simulink model "Basics"  (R2019a)
settings: Solver=ode1  StartTime=0.0  StopTime=2.5  FixedStep=Ts_Power  RelTol=1e-3
PostLoadFcn:
  | %% Init for wind PnO models - global system parameters
  | OVERRIDE_SSN_MEMORY_LIMIT=1;
  | Ts=50e-6;
  | % Ts=50e-10;
  | Ts_Power=Ts;
  | Ts_Control=2*Ts;
  | freq = 50;
  | Fnom=freq;
  | Vac=400e3;
InitFcn:
  | %% Init for wind PnO models - global system parameters
  | OVERRIDE_SSN_MEMORY_LIMIT=1;
  | Ts=50e-6;
  | % Ts=50e-10;
  | Ts_Power=Ts;
  | Ts_Control=2*Ts;
  | freq = 50;
  | Fnom=freq;
  | Vac=225e3;
values from neighbouring files (symbols this model uses):
  ohl_posCap = 11.33e-009/2    (= 5.665e-09)    [variable.m]
  ohl_posInd = 1.05e-3/2    (= 0.000525)    [variable.m]
  ohl_posR = 0.1153/2    (= 0.05765)    [variable.m]
  ohl_zeroCap = 5.01e-009/2    (= 2.505e-09)    [variable.m]
  ohl_zeroInd = 3.32e-3/2    (= 0.00166)    [variable.m]
  ohl_zeroR = 0.4138/2    (= 0.2069)    [variable.m]
  sub_posCap = 0.16e-006    (= 1.6e-07)    [variable.m]
  sub_posInd = 0.001400563    [variable.m]
  sub_posR = 0.036    [variable.m]
  sub_zeroCap = 0.053333e-006    (= 5.3333e-08)    [variable.m]
  sub_zeroInd = 0.00420169    [variable.m]
  sub_zeroR = 0.108    [variable.m]
  transfo_L1 = 0.05999374    [variable.m]
  transfo_L2 = 0.05999374    [variable.m]
  transfo_R1 = 0.000866667    [variable.m]
  transfo_R2 = 0.00086667    [variable.m]
undefined symbols (not defined in the file or in its folder): D1, D11, Delta, den, DiscIntNeverNeededParam, dx, find_system, gcbh, num, out_Buses, out_WindFarms, sps_rtmsupport
libraries: powerlib x173, simulink x80, powerlib_meascontrol x80, elements x52, eeSinusoidalMeasurement x46, simulink_extras x40, spsVIMeasurementModel x36, eePowerMeasurement x15
(part 14 of 22)

== system Basics/SM_WT1/Differential Element 1/Main Protection (Current Differential)/Charging Current Compensation phase A/DAB7 ==
  a : Inport
  AD & Buffer : S-Function  FunctionName=dab2  Parameters=winsize,fs,dx,resdis  SFunctionDeploymentMode=off  EnableBusSupport=off
  Analog Filter : TransferFcn  Numerator=num  Denominator=den
  Gain : Gain  Gain=G  SaturateOnIntegerOverflow=on  OutDataTypeStr=Inherit: Same as input  ParamDataTypeStr=Inherit: Same as input
  Zero-Order Hold : ZeroOrderHold  SampleTime=1/fs
  d : Outport  InitialOutput=[zeros(winsize,1)]  VectorParamsAs1DForOutWhenUnconnected=on
  wires:
  AD & Buffer/1 -> d/1
  a/1 -> Analog Filter/1
  Zero-Order Hold/1 -> AD & Buffer/1
  Gain/1 -> Zero-Order Hold/1
  Analog Filter/1 -> Gain/1

== system Basics/SM_WT1/Differential Element 1/Main Protection (Current Differential)/Charging Current Compensation phase B/DAB5 ==
  a : Inport
  AD & Buffer : S-Function  FunctionName=dab2  Parameters=winsize,fs,dx,resdis  SFunctionDeploymentMode=off  EnableBusSupport=off
  Analog Filter : TransferFcn  Numerator=num  Denominator=den
  Gain : Gain  Gain=G  SaturateOnIntegerOverflow=on  OutDataTypeStr=Inherit: Same as input  ParamDataTypeStr=Inherit: Same as input
  Zero-Order Hold : ZeroOrderHold  SampleTime=1/fs
  d : Outport  InitialOutput=[zeros(winsize,1)]  VectorParamsAs1DForOutWhenUnconnected=on
  wires:
  AD & Buffer/1 -> d/1
  a/1 -> Analog Filter/1
  Zero-Order Hold/1 -> AD & Buffer/1
  Gain/1 -> Zero-Order Hold/1
  Analog Filter/1 -> Gain/1

== system Basics/SM_WT1/Differential Element 1/Main Protection (Current Differential)/Charging Current Compensation phase B/DAB6 ==
  a : Inport
  AD & Buffer : S-Function  FunctionName=dab2  Parameters=winsize,fs,dx,resdis  SFunctionDeploymentMode=off  EnableBusSupport=off
  Analog Filter : TransferFcn  Numerator=num  Denominator=den
  Gain : Gain  Gain=G  SaturateOnIntegerOverflow=on  OutDataTypeStr=Inherit: Same as input  ParamDataTypeStr=Inherit: Same as input
  Zero-Order Hold : ZeroOrderHold  SampleTime=1/fs
  d : Outport  InitialOutput=[zeros(winsize,1)]  VectorParamsAs1DForOutWhenUnconnected=on
  wires:
  Analog Filter/1 -> Gain/1
  Gain/1 -> Zero-Order Hold/1
  Zero-Order Hold/1 -> AD & Buffer/1
  a/1 -> Analog Filter/1
  AD & Buffer/1 -> d/1

== system Basics/SM_WT1/Differential Element 1/Main Protection (Current Differential)/Charging Current Compensation phase B/DAB7 ==
  a : Inport
  AD & Buffer : S-Function  FunctionName=dab2  Parameters=winsize,fs,dx,resdis  SFunctionDeploymentMode=off  EnableBusSupport=off
  Analog Filter : TransferFcn  Numerator=num  Denominator=den
  Gain : Gain  Gain=G  SaturateOnIntegerOverflow=on  OutDataTypeStr=Inherit: Same as input  ParamDataTypeStr=Inherit: Same as input
  Zero-Order Hold : ZeroOrderHold  SampleTime=1/fs
  d : Outport  InitialOutput=[zeros(winsize,1)]  VectorParamsAs1DForOutWhenUnconnected=on
  wires:
  AD & Buffer/1 -> d/1
  a/1 -> Analog Filter/1
  Zero-Order Hold/1 -> AD & Buffer/1
  Gain/1 -> Zero-Order Hold/1
  Analog Filter/1 -> Gain/1

== system Basics/SM_WT1/Differential Element 1/Main Protection (Current Differential)/Charging Current Compensation phase C/DAB5 ==
  a : Inport
  AD & Buffer : S-Function  FunctionName=dab2  Parameters=winsize,fs,dx,resdis  SFunctionDeploymentMode=off  EnableBusSupport=off
  Analog Filter : TransferFcn  Numerator=num  Denominator=den
  Gain : Gain  Gain=G  SaturateOnIntegerOverflow=on  OutDataTypeStr=Inherit: Same as input  ParamDataTypeStr=Inherit: Same as input
  Zero-Order Hold : ZeroOrderHold  SampleTime=1/fs
  d : Outport  InitialOutput=[zeros(winsize,1)]  VectorParamsAs1DForOutWhenUnconnected=on
  wires:
  AD & Buffer/1 -> d/1
  a/1 -> Analog Filter/1
  Zero-Order Hold/1 -> AD & Buffer/1
  Gain/1 -> Zero-Order Hold/1
  Analog Filter/1 -> Gain/1

== system Basics/SM_WT1/Differential Element 1/Main Protection (Current Differential)/Charging Current Compensation phase C/DAB6 ==
  a : Inport
  AD & Buffer : S-Function  FunctionName=dab2  Parameters=winsize,fs,dx,resdis  SFunctionDeploymentMode=off  EnableBusSupport=off
  Analog Filter : TransferFcn  Numerator=num  Denominator=den
  Gain : Gain  Gain=G  SaturateOnIntegerOverflow=on  OutDataTypeStr=Inherit: Same as input  ParamDataTypeStr=Inherit: Same as input
  Zero-Order Hold : ZeroOrderHold  SampleTime=1/fs
  d : Outport  InitialOutput=[zeros(winsize,1)]  VectorParamsAs1DForOutWhenUnconnected=on
  wires:
  Analog Filter/1 -> Gain/1
  Gain/1 -> Zero-Order Hold/1
  Zero-Order Hold/1 -> AD & Buffer/1
  a/1 -> Analog Filter/1
  AD & Buffer/1 -> d/1

== system Basics/SM_WT1/Differential Element 1/Main Protection (Current Differential)/Charging Current Compensation phase C/DAB7 ==
  a : Inport
  AD & Buffer : S-Function  FunctionName=dab2  Parameters=winsize,fs,dx,resdis  SFunctionDeploymentMode=off  EnableBusSupport=off
  Analog Filter : TransferFcn  Numerator=num  Denominator=den
  Gain : Gain  Gain=G  SaturateOnIntegerOverflow=on  OutDataTypeStr=Inherit: Same as input  ParamDataTypeStr=Inherit: Same as input
  Zero-Order Hold : ZeroOrderHold  SampleTime=1/fs
  d : Outport  InitialOutput=[zeros(winsize,1)]  VectorParamsAs1DForOutWhenUnconnected=on
  wires:
  AD & Buffer/1 -> d/1
  a/1 -> Analog Filter/1
  Zero-Order Hold/1 -> AD & Buffer/1
  Gain/1 -> Zero-Order Hold/1
  Analog Filter/1 -> Gain/1

== system Basics/SM_WT1/Differential Element 1/Main Protection (Current Differential)/Current Differential Protection for Phase A/Comparision Scheme ==
  I_Slave : Inport
  I_Master : Inport  Port=2
  Abs : Abs  SaturateOnIntegerOverflow=on
  Abs1 : Abs  SaturateOnIntegerOverflow=on
  Bias Characteristic1 : elements/Bias Characteristic  BC=bias  fs=Freq*20
  "Differential Current " : Sum  SaturateOnIntegerOverflow=on  InputSameDT=on  OutDataTypeStr=Inherit: Same as first input
  Restraining Current : Sum  Inputs=+-  SaturateOnIntegerOverflow=on  InputSameDT=on  OutDataTypeStr=Inherit: Same as first input
  Pickup : Outport  VectorParamsAs1DForOutWhenUnconnected=on
  wires:
  "Differential Current "/1 -> Abs/1
  Abs1/1 -> Bias Characteristic1/2
  Bias Characteristic1/1 -> Pickup/1
  Abs/1 -> Bias Characteristic1/1
  I_Master/1 -> Restraining Current/2, "Differential Current "/2
  I_Slave/1 -> Restraining Current/1, "Differential Current "/1
  Restraining Current/1 -> Abs1/1

== system Basics/SM_WT1/Differential Element 1/Main Protection (Current Differential)/Current Differential Protection for Phase A/DAB4 ==
  a : Inport
  AD & Buffer : S-Function  FunctionName=dab2  Parameters=winsize,fs,dx,resdis  SFunctionDeploymentMode=off  EnableBusSupport=off
  Analog Filter : TransferFcn  Numerator=num  Denominator=den
  Gain : Gain  Gain=G  SaturateOnIntegerOverflow=on  OutDataTypeStr=Inherit: Same as input  ParamDataTypeStr=Inherit: Same as input
  Zero-Order Hold : ZeroOrderHold  SampleTime=1/fs
  d : Outport  InitialOutput=[zeros(winsize,1)]  VectorParamsAs1DForOutWhenUnconnected=on
  wires:
  AD & Buffer/1 -> d/1
  a/1 -> Analog Filter/1
  Zero-Order Hold/1 -> AD & Buffer/1
  Gain/1 -> Zero-Order Hold/1
  Analog Filter/1 -> Gain/1

== system Basics/SM_WT1/Differential Element 1/Main Protection (Current Differential)/Current Differential Protection for Phase A/DAB8 ==
  a : Inport
  AD & Buffer : S-Function  FunctionName=dab2  Parameters=winsize,fs,dx,resdis  SFunctionDeploymentMode=off  EnableBusSupport=off
  Analog Filter : TransferFcn  Numerator=num  Denominator=den
  Gain : Gain  Gain=G  SaturateOnIntegerOverflow=on  OutDataTypeStr=Inherit: Same as input  ParamDataTypeStr=Inherit: Same as input
  Zero-Order Hold : ZeroOrderHold  SampleTime=1/fs
  d : Outport  InitialOutput=[zeros(winsize,1)]  VectorParamsAs1DForOutWhenUnconnected=on
  wires:
  Analog Filter/1 -> Gain/1
  Gain/1 -> Zero-Order Hold/1
  Zero-Order Hold/1 -> AD & Buffer/1
  a/1 -> Analog Filter/1
  AD & Buffer/1 -> d/1

== system Basics/SM_WT1/Differential Element 1/Main Protection (Current Differential)/Current Differential Protection for Phase B/Comparision Scheme ==
  I_Slave : Inport
  I_Master : Inport  Port=2
  Abs : Abs  SaturateOnIntegerOverflow=on
  Abs1 : Abs  SaturateOnIntegerOverflow=on
  Bias Characteristic1 : elements/Bias Characteristic  BC=bias  fs=Freq*20
  "Differential Current " : Sum  SaturateOnIntegerOverflow=on  InputSameDT=on  OutDataTypeStr=Inherit: Same as first input
  Restraining Current : Sum  Inputs=+-  SaturateOnIntegerOverflow=on  InputSameDT=on  OutDataTypeStr=Inherit: Same as first input
  Pickup : Outport  VectorParamsAs1DForOutWhenUnconnected=on
  wires:
  Restraining Current/1 -> Abs1/1
  I_Slave/1 -> "Differential Current "/1, Restraining Current/1
  I_Master/1 -> "Differential Current "/2, Restraining Current/2
  Abs/1 -> Bias Characteristic1/1
  Bias Characteristic1/1 -> Pickup/1
  Abs1/1 -> Bias Characteristic1/2
  "Differential Current "/1 -> Abs/1

== system Basics/SM_WT1/Differential Element 1/Main Protection (Current Differential)/Current Differential Protection for Phase B/DAB4 ==
  a : Inport
  AD & Buffer : S-Function  FunctionName=dab2  Parameters=winsize,fs,dx,resdis  SFunctionDeploymentMode=off  EnableBusSupport=off
  Analog Filter : TransferFcn  Numerator=num  Denominator=den
  Gain : Gain  Gain=G  SaturateOnIntegerOverflow=on  OutDataTypeStr=Inherit: Same as input  ParamDataTypeStr=Inherit: Same as input
  Zero-Order Hold : ZeroOrderHold  SampleTime=1/fs
  d : Outport  InitialOutput=[zeros(winsize,1)]  VectorParamsAs1DForOutWhenUnconnected=on
  wires:
  Analog Filter/1 -> Gain/1
  Gain/1 -> Zero-Order Hold/1
  Zero-Order Hold/1 -> AD & Buffer/1
  a/1 -> Analog Filter/1
  AD & Buffer/1 -> d/1

== system Basics/SM_WT1/Differential Element 1/Main Protection (Current Differential)/Current Differential Protection for Phase B/DAB8 ==
  a : Inport
  AD & Buffer : S-Function  FunctionName=dab2  Parameters=winsize,fs,dx,resdis  SFunctionDeploymentMode=off  EnableBusSupport=off
  Analog Filter : TransferFcn  Numerator=num  Denominator=den
  Gain : Gain  Gain=G  SaturateOnIntegerOverflow=on  OutDataTypeStr=Inherit: Same as input  ParamDataTypeStr=Inherit: Same as input
  Zero-Order Hold : ZeroOrderHold  SampleTime=1/fs
  d : Outport  InitialOutput=[zeros(winsize,1)]  VectorParamsAs1DForOutWhenUnconnected=on
  wires:
  AD & Buffer/1 -> d/1
  a/1 -> Analog Filter/1
  Zero-Order Hold/1 -> AD & Buffer/1
  Gain/1 -> Zero-Order Hold/1
  Analog Filter/1 -> Gain/1

== system Basics/SM_WT1/Differential Element 1/Main Protection (Current Differential)/Current Differential Protection for Phase C/Comparision Scheme ==
  I_Slave : Inport
  I_Master : Inport  Port=2
  Abs : Abs  SaturateOnIntegerOverflow=on
  Abs1 : Abs  SaturateOnIntegerOverflow=on
  Bias Characteristic1 : elements/Bias Characteristic  BC=bias  fs=Freq*20
  "Differential Current " : Sum  SaturateOnIntegerOverflow=on  InputSameDT=on  OutDataTypeStr=Inherit: Same as first input
  Restraining Current : Sum  Inputs=+-  SaturateOnIntegerOverflow=on  InputSameDT=on  OutDataTypeStr=Inherit: Same as first input
  Pickup : Outport  VectorParamsAs1DForOutWhenUnconnected=on
  wires:
  "Differential Current "/1 -> Abs/1
  Abs1/1 -> Bias Characteristic1/2
  Bias Characteristic1/1 -> Pickup/1
  Abs/1 -> Bias Characteristic1/1
  I_Master/1 -> Restraining Current/2, "Differential Current "/2
  I_Slave/1 -> Restraining Current/1, "Differential Current "/1
  Restraining Current/1 -> Abs1/1

== system Basics/SM_WT1/Differential Element 1/Main Protection (Current Differential)/Current Differential Protection for Phase C/DAB4 ==
  a : Inport
  AD & Buffer : S-Function  FunctionName=dab2  Parameters=winsize,fs,dx,resdis  SFunctionDeploymentMode=off  EnableBusSupport=off
  Analog Filter : TransferFcn  Numerator=num  Denominator=den
  Gain : Gain  Gain=G  SaturateOnIntegerOverflow=on  OutDataTypeStr=Inherit: Same as input  ParamDataTypeStr=Inherit: Same as input
  Zero-Order Hold : ZeroOrderHold  SampleTime=1/fs
  d : Outport  InitialOutput=[zeros(winsize,1)]  VectorParamsAs1DForOutWhenUnconnected=on
  wires:
  AD & Buffer/1 -> d/1
  a/1 -> Analog Filter/1
  Zero-Order Hold/1 -> AD & Buffer/1
  Gain/1 -> Zero-Order Hold/1
  Analog Filter/1 -> Gain/1

== system Basics/SM_WT1/Differential Element 1/Main Protection (Current Differential)/Current Differential Protection for Phase C/DAB8 ==
  a : Inport
  AD & Buffer : S-Function  FunctionName=dab2  Parameters=winsize,fs,dx,resdis  SFunctionDeploymentMode=off  EnableBusSupport=off
  Analog Filter : TransferFcn  Numerator=num  Denominator=den
  Gain : Gain  Gain=G  SaturateOnIntegerOverflow=on  OutDataTypeStr=Inherit: Same as input  ParamDataTypeStr=Inherit: Same as input
  Zero-Order Hold : ZeroOrderHold  SampleTime=1/fs
  d : Outport  InitialOutput=[zeros(winsize,1)]  VectorParamsAs1DForOutWhenUnconnected=on
  wires:
  Analog Filter/1 -> Gain/1
  Gain/1 -> Zero-Order Hold/1
  Zero-Order Hold/1 -> AD & Buffer/1
  a/1 -> Analog Filter/1
  AD & Buffer/1 -> d/1

== system Basics/SM_WT1/Differential Element 2/Main Protection (Current Differential)/Charging Current Compensation phase A/DAB5 ==
  a : Inport
  AD & Buffer : S-Function  FunctionName=dab2  Parameters=winsize,fs,dx,resdis  SFunctionDeploymentMode=off  EnableBusSupport=off
  Analog Filter : TransferFcn  Numerator=num  Denominator=den
  Gain : Gain  Gain=G  SaturateOnIntegerOverflow=on  OutDataTypeStr=Inherit: Same as input  ParamDataTypeStr=Inherit: Same as input
  Zero-Order Hold : ZeroOrderHold  SampleTime=1/fs
  d : Outport  InitialOutput=[zeros(winsize,1)]  VectorParamsAs1DForOutWhenUnconnected=on
  wires:
  AD & Buffer/1 -> d/1
  a/1 -> Analog Filter/1
  Zero-Order Hold/1 -> AD & Buffer/1
  Gain/1 -> Zero-Order Hold/1
  Analog Filter/1 -> Gain/1

== system Basics/SM_WT1/Differential Element 2/Main Protection (Current Differential)/Charging Current Compensation phase A/DAB6 ==
  a : Inport
  AD & Buffer : S-Function  FunctionName=dab2  Parameters=winsize,fs,dx,resdis  SFunctionDeploymentMode=off  EnableBusSupport=off
  Analog Filter : TransferFcn  Numerator=num  Denominator=den
  Gain : Gain  Gain=G  SaturateOnIntegerOverflow=on  OutDataTypeStr=Inherit: Same as input  ParamDataTypeStr=Inherit: Same as input
  Zero-Order Hold : ZeroOrderHold  SampleTime=1/fs
  d : Outport  InitialOutput=[zeros(winsize,1)]  VectorParamsAs1DForOutWhenUnconnected=on
  wires:
  Analog Filter/1 -> Gain/1
  Gain/1 -> Zero-Order Hold/1
  Zero-Order Hold/1 -> AD & Buffer/1
  a/1 -> Analog Filter/1
  AD & Buffer/1 -> d/1

== system Basics/SM_WT1/Differential Element 2/Main Protection (Current Differential)/Charging Current Compensation phase A/DAB7 ==
  a : Inport
  AD & Buffer : S-Function  FunctionName=dab2  Parameters=winsize,fs,dx,resdis  SFunctionDeploymentMode=off  EnableBusSupport=off
  Analog Filter : TransferFcn  Numerator=num  Denominator=den
  Gain : Gain  Gain=G  SaturateOnIntegerOverflow=on  OutDataTypeStr=Inherit: Same as input  ParamDataTypeStr=Inherit: Same as input
  Zero-Order Hold : ZeroOrderHold  SampleTime=1/fs
  d : Outport  InitialOutput=[zeros(winsize,1)]  VectorParamsAs1DForOutWhenUnconnected=on
  wires:
  AD & Buffer/1 -> d/1
  a/1 -> Analog Filter/1
  Zero-Order Hold/1 -> AD & Buffer/1
  Gain/1 -> Zero-Order Hold/1
  Analog Filter/1 -> Gain/1

== system Basics/SM_WT1/Differential Element 2/Main Protection (Current Differential)/Charging Current Compensation phase B/DAB5 ==
  a : Inport
  AD & Buffer : S-Function  FunctionName=dab2  Parameters=winsize,fs,dx,resdis  SFunctionDeploymentMode=off  EnableBusSupport=off
  Analog Filter : TransferFcn  Numerator=num  Denominator=den
  Gain : Gain  Gain=G  SaturateOnIntegerOverflow=on  OutDataTypeStr=Inherit: Same as input  ParamDataTypeStr=Inherit: Same as input
  Zero-Order Hold : ZeroOrderHold  SampleTime=1/fs
  d : Outport  InitialOutput=[zeros(winsize,1)]  VectorParamsAs1DForOutWhenUnconnected=on
  wires:
  AD & Buffer/1 -> d/1
  a/1 -> Analog Filter/1
  Zero-Order Hold/1 -> AD & Buffer/1
  Gain/1 -> Zero-Order Hold/1
  Analog Filter/1 -> Gain/1

== system Basics/SM_WT1/Differential Element 2/Main Protection (Current Differential)/Charging Current Compensation phase B/DAB6 ==
  a : Inport
  AD & Buffer : S-Function  FunctionName=dab2  Parameters=winsize,fs,dx,resdis  SFunctionDeploymentMode=off  EnableBusSupport=off
  Analog Filter : TransferFcn  Numerator=num  Denominator=den
  Gain : Gain  Gain=G  SaturateOnIntegerOverflow=on  OutDataTypeStr=Inherit: Same as input  ParamDataTypeStr=Inherit: Same as input
  Zero-Order Hold : ZeroOrderHold  SampleTime=1/fs
  d : Outport  InitialOutput=[zeros(winsize,1)]  VectorParamsAs1DForOutWhenUnconnected=on
  wires:
  Analog Filter/1 -> Gain/1
  Gain/1 -> Zero-Order Hold/1
  Zero-Order Hold/1 -> AD & Buffer/1
  a/1 -> Analog Filter/1
  AD & Buffer/1 -> d/1

== system Basics/SM_WT1/Differential Element 2/Main Protection (Current Differential)/Charging Current Compensation phase B/DAB7 ==
  a : Inport
  AD & Buffer : S-Function  FunctionName=dab2  Parameters=winsize,fs,dx,resdis  SFunctionDeploymentMode=off  EnableBusSupport=off
  Analog Filter : TransferFcn  Numerator=num  Denominator=den
  Gain : Gain  Gain=G  SaturateOnIntegerOverflow=on  OutDataTypeStr=Inherit: Same as input  ParamDataTypeStr=Inherit: Same as input
  Zero-Order Hold : ZeroOrderHold  SampleTime=1/fs
  d : Outport  InitialOutput=[zeros(winsize,1)]  VectorParamsAs1DForOutWhenUnconnected=on
  wires:
  AD & Buffer/1 -> d/1
  a/1 -> Analog Filter/1
  Zero-Order Hold/1 -> AD & Buffer/1
  Gain/1 -> Zero-Order Hold/1
  Analog Filter/1 -> Gain/1

== system Basics/SM_WT1/Differential Element 2/Main Protection (Current Differential)/Charging Current Compensation phase C/DAB5 ==
  a : Inport
  AD & Buffer : S-Function  FunctionName=dab2  Parameters=winsize,fs,dx,resdis  SFunctionDeploymentMode=off  EnableBusSupport=off
  Analog Filter : TransferFcn  Numerator=num  Denominator=den
  Gain : Gain  Gain=G  SaturateOnIntegerOverflow=on  OutDataTypeStr=Inherit: Same as input  ParamDataTypeStr=Inherit: Same as input
  Zero-Order Hold : ZeroOrderHold  SampleTime=1/fs
  d : Outport  InitialOutput=[zeros(winsize,1)]  VectorParamsAs1DForOutWhenUnconnected=on
  wires:
  AD & Buffer/1 -> d/1
  a/1 -> Analog Filter/1
  Zero-Order Hold/1 -> AD & Buffer/1
  Gain/1 -> Zero-Order Hold/1
  Analog Filter/1 -> Gain/1

== system Basics/SM_WT1/Differential Element 2/Main Protection (Current Differential)/Charging Current Compensation phase C/DAB6 ==
  a : Inport
  AD & Buffer : S-Function  FunctionName=dab2  Parameters=winsize,fs,dx,resdis  SFunctionDeploymentMode=off  EnableBusSupport=off
  Analog Filter : TransferFcn  Numerator=num  Denominator=den
  Gain : Gain  Gain=G  SaturateOnIntegerOverflow=on  OutDataTypeStr=Inherit: Same as input  ParamDataTypeStr=Inherit: Same as input
  Zero-Order Hold : ZeroOrderHold  SampleTime=1/fs
  d : Outport  InitialOutput=[zeros(winsize,1)]  VectorParamsAs1DForOutWhenUnconnected=on
  wires:
  Analog Filter/1 -> Gain/1
  Gain/1 -> Zero-Order Hold/1
  Zero-Order Hold/1 -> AD & Buffer/1
  a/1 -> Analog Filter/1
  AD & Buffer/1 -> d/1

== system Basics/SM_WT1/Differential Element 2/Main Protection (Current Differential)/Charging Current Compensation phase C/DAB7 ==
  a : Inport
  AD & Buffer : S-Function  FunctionName=dab2  Parameters=winsize,fs,dx,resdis  SFunctionDeploymentMode=off  EnableBusSupport=off
  Analog Filter : TransferFcn  Numerator=num  Denominator=den
  Gain : Gain  Gain=G  SaturateOnIntegerOverflow=on  OutDataTypeStr=Inherit: Same as input  ParamDataTypeStr=Inherit: Same as input
  Zero-Order Hold : ZeroOrderHold  SampleTime=1/fs
  d : Outport  InitialOutput=[zeros(winsize,1)]  VectorParamsAs1DForOutWhenUnconnected=on
  wires:
  AD & Buffer/1 -> d/1
  a/1 -> Analog Filter/1
  Zero-Order Hold/1 -> AD & Buffer/1
  Gain/1 -> Zero-Order Hold/1
  Analog Filter/1 -> Gain/1

== system Basics/SM_WT1/Differential Element 2/Main Protection (Current Differential)/Current Differential Protection for Phase A/Comparision Scheme ==
  I_Slave : Inport
  I_Master : Inport  Port=2
  Abs : Abs  SaturateOnIntegerOverflow=on
  Abs1 : Abs  SaturateOnIntegerOverflow=on
  Bias Characteristic1 : elements/Bias Characteristic  BC=bias  fs=Freq*20
  "Differential Current " : Sum  SaturateOnIntegerOverflow=on  InputSameDT=on  OutDataTypeStr=Inherit: Same as first input
  Restraining Current : Sum  Inputs=+-  SaturateOnIntegerOverflow=on  InputSameDT=on  OutDataTypeStr=Inherit: Same as first input
  Pickup : Outport  VectorParamsAs1DForOutWhenUnconnected=on
  wires:
  "Differential Current "/1 -> Abs/1
  Abs1/1 -> Bias Characteristic1/2
  Bias Characteristic1/1 -> Pickup/1
  Abs/1 -> Bias Characteristic1/1
  I_Master/1 -> Restraining Current/2, "Differential Current "/2
  I_Slave/1 -> Restraining Current/1, "Differential Current "/1
  Restraining Current/1 -> Abs1/1

== system Basics/SM_WT1/Differential Element 2/Main Protection (Current Differential)/Current Differential Protection for Phase A/DAB4 ==
  a : Inport
  AD & Buffer : S-Function  FunctionName=dab2  Parameters=winsize,fs,dx,resdis  SFunctionDeploymentMode=off  EnableBusSupport=off
  Analog Filter : TransferFcn  Numerator=num  Denominator=den
  Gain : Gain  Gain=G  SaturateOnIntegerOverflow=on  OutDataTypeStr=Inherit: Same as input  ParamDataTypeStr=Inherit: Same as input
  Zero-Order Hold : ZeroOrderHold  SampleTime=1/fs
  d : Outport  InitialOutput=[zeros(winsize,1)]  VectorParamsAs1DForOutWhenUnconnected=on
  wires:
  AD & Buffer/1 -> d/1
  a/1 -> Analog Filter/1
  Zero-Order Hold/1 -> AD & Buffer/1
  Gain/1 -> Zero-Order Hold/1
  Analog Filter/1 -> Gain/1

== system Basics/SM_WT1/Differential Element 2/Main Protection (Current Differential)/Current Differential Protection for Phase A/DAB8 ==
  a : Inport
  AD & Buffer : S-Function  FunctionName=dab2  Parameters=winsize,fs,dx,resdis  SFunctionDeploymentMode=off  EnableBusSupport=off
  Analog Filter : TransferFcn  Numerator=num  Denominator=den
  Gain : Gain  Gain=G  SaturateOnIntegerOverflow=on  OutDataTypeStr=Inherit: Same as input  ParamDataTypeStr=Inherit: Same as input
  Zero-Order Hold : ZeroOrderHold  SampleTime=1/fs
  d : Outport  InitialOutput=[zeros(winsize,1)]  VectorParamsAs1DForOutWhenUnconnected=on
  wires:
  Analog Filter/1 -> Gain/1
  Gain/1 -> Zero-Order Hold/1
  Zero-Order Hold/1 -> AD & Buffer/1
  a/1 -> Analog Filter/1
  AD & Buffer/1 -> d/1

== system Basics/SM_WT1/Differential Element 2/Main Protection (Current Differential)/Current Differential Protection for Phase B/Comparision Scheme ==
  I_Slave : Inport
  I_Master : Inport  Port=2
  Abs : Abs  SaturateOnIntegerOverflow=on
  Abs1 : Abs  SaturateOnIntegerOverflow=on
  Bias Characteristic1 : elements/Bias Characteristic  BC=bias  fs=Freq*20
  "Differential Current " : Sum  SaturateOnIntegerOverflow=on  InputSameDT=on  OutDataTypeStr=Inherit: Same as first input
  Restraining Current : Sum  Inputs=+-  SaturateOnIntegerOverflow=on  InputSameDT=on  OutDataTypeStr=Inherit: Same as first input
  Pickup : Outport  VectorParamsAs1DForOutWhenUnconnected=on
  wires:
  Restraining Current/1 -> Abs1/1
  I_Slave/1 -> "Differential Current "/1, Restraining Current/1
  I_Master/1 -> "Differential Current "/2, Restraining Current/2
  Abs/1 -> Bias Characteristic1/1
  Bias Characteristic1/1 -> Pickup/1
  Abs1/1 -> Bias Characteristic1/2
  "Differential Current "/1 -> Abs/1

== system Basics/SM_WT1/Differential Element 2/Main Protection (Current Differential)/Current Differential Protection for Phase B/DAB4 ==
  a : Inport
  AD & Buffer : S-Function  FunctionName=dab2  Parameters=winsize,fs,dx,resdis  SFunctionDeploymentMode=off  EnableBusSupport=off
  Analog Filter : TransferFcn  Numerator=num  Denominator=den
  Gain : Gain  Gain=G  SaturateOnIntegerOverflow=on  OutDataTypeStr=Inherit: Same as input  ParamDataTypeStr=Inherit: Same as input
  Zero-Order Hold : ZeroOrderHold  SampleTime=1/fs
  d : Outport  InitialOutput=[zeros(winsize,1)]  VectorParamsAs1DForOutWhenUnconnected=on
  wires:
  Analog Filter/1 -> Gain/1
  Gain/1 -> Zero-Order Hold/1
  Zero-Order Hold/1 -> AD & Buffer/1
  a/1 -> Analog Filter/1
  AD & Buffer/1 -> d/1

== system Basics/SM_WT1/Differential Element 2/Main Protection (Current Differential)/Current Differential Protection for Phase B/DAB8 ==
  a : Inport
  AD & Buffer : S-Function  FunctionName=dab2  Parameters=winsize,fs,dx,resdis  SFunctionDeploymentMode=off  EnableBusSupport=off
  Analog Filter : TransferFcn  Numerator=num  Denominator=den
  Gain : Gain  Gain=G  SaturateOnIntegerOverflow=on  OutDataTypeStr=Inherit: Same as input  ParamDataTypeStr=Inherit: Same as input
  Zero-Order Hold : ZeroOrderHold  SampleTime=1/fs
  d : Outport  InitialOutput=[zeros(winsize,1)]  VectorParamsAs1DForOutWhenUnconnected=on
  wires:
  AD & Buffer/1 -> d/1
  a/1 -> Analog Filter/1
  Zero-Order Hold/1 -> AD & Buffer/1
  Gain/1 -> Zero-Order Hold/1
  Analog Filter/1 -> Gain/1

== system Basics/SM_WT1/Differential Element 2/Main Protection (Current Differential)/Current Differential Protection for Phase C/Comparision Scheme ==
  I_Slave : Inport
  I_Master : Inport  Port=2
  Abs : Abs  SaturateOnIntegerOverflow=on
  Abs1 : Abs  SaturateOnIntegerOverflow=on
  Bias Characteristic1 : elements/Bias Characteristic  BC=bias  fs=Freq*20
  "Differential Current " : Sum  SaturateOnIntegerOverflow=on  InputSameDT=on  OutDataTypeStr=Inherit: Same as first input
  Restraining Current : Sum  Inputs=+-  SaturateOnIntegerOverflow=on  InputSameDT=on  OutDataTypeStr=Inherit: Same as first input
  Pickup : Outport  VectorParamsAs1DForOutWhenUnconnected=on
  wires:
  "Differential Current "/1 -> Abs/1
  Abs1/1 -> Bias Characteristic1/2
  Bias Characteristic1/1 -> Pickup/1
  Abs/1 -> Bias Characteristic1/1
  I_Master/1 -> Restraining Current/2, "Differential Current "/2
  I_Slave/1 -> Restraining Current/1, "Differential Current "/1
  Restraining Current/1 -> Abs1/1

== system Basics/SM_WT1/Differential Element 2/Main Protection (Current Differential)/Current Differential Protection for Phase C/DAB4 ==
  a : Inport
  AD & Buffer : S-Function  FunctionName=dab2  Parameters=winsize,fs,dx,resdis  SFunctionDeploymentMode=off  EnableBusSupport=off
  Analog Filter : TransferFcn  Numerator=num  Denominator=den
  Gain : Gain  Gain=G  SaturateOnIntegerOverflow=on  OutDataTypeStr=Inherit: Same as input  ParamDataTypeStr=Inherit: Same as input
  Zero-Order Hold : ZeroOrderHold  SampleTime=1/fs
  d : Outport  InitialOutput=[zeros(winsize,1)]  VectorParamsAs1DForOutWhenUnconnected=on
  wires:
  AD & Buffer/1 -> d/1
  a/1 -> Analog Filter/1
  Zero-Order Hold/1 -> AD & Buffer/1
  Gain/1 -> Zero-Order Hold/1
  Analog Filter/1 -> Gain/1

== system Basics/SM_WT1/Differential Element 2/Main Protection (Current Differential)/Current Differential Protection for Phase C/DAB8 ==
  a : Inport
  AD & Buffer : S-Function  FunctionName=dab2  Parameters=winsize,fs,dx,resdis  SFunctionDeploymentMode=off  EnableBusSupport=off
  Analog Filter : TransferFcn  Numerator=num  Denominator=den
  Gain : Gain  Gain=G  SaturateOnIntegerOverflow=on  OutDataTypeStr=Inherit: Same as input  ParamDataTypeStr=Inherit: Same as input
  Zero-Order Hold : ZeroOrderHold  SampleTime=1/fs
  d : Outport  InitialOutput=[zeros(winsize,1)]  VectorParamsAs1DForOutWhenUnconnected=on
  wires:
  Analog Filter/1 -> Gain/1
  Gain/1 -> Zero-Order Hold/1
  Zero-Order Hold/1 -> AD & Buffer/1
  a/1 -> Analog Filter/1
  AD & Buffer/1 -> d/1

== system Basics/SM_WT1/Impedance Element 1/Impedance Relay Scheme/Analog filtering, signal conditioning/CURRENTS ==
  Iabc : Inport
  Add : Sum  Inputs=+++
  Complex{,1..3} (4 alike) : MagnitudeAngleToComplex
  Constant : Constant  Value=pi/180
  Constant1 : Constant  Value=k0m1
  Constant2 : Constant  Value=k0a1
  DAB - current A : Subsystem  AncestorBlock=elements/DAB  mask(Data Adquisition Board){filter=off, approx=Butterworth, order=2, numerator=[], denominator=[], freq=fCut, resdis=off, vertres=16, xmax=CurrentRange, winsize=WindowSize, G=1.0, fs=fSampling}
      mask prompts: filter "Disable Analog Filter"; approx "Filter approximation"; numerator "Free expression filter: numerator(descending order of s)"; denominator "Free expression filter: denominator:"; freq "Cut-off frequency"; resdis "Disable Vertical Resolution"; vertres "Vertical Resolution: No. of bits"; xmax "Vertical Resolution: signal range"; winsize "Window size"; G "Gain"; fs "Sampling frequency"
      mask help: Performs analog filtering, signal conditioning and sampling. A single signal is the input, a buffer with the signal samples is the output. The options include analog filter enable/disable switch, type, order and cut-off frequency of the analog filter, conditioning gain, sampling frequency, number of bits, the length of the buffer.
      mask init:
      | dab1
      mask Help: web(['file:///' which('dabdoc2.html')]);
      mask TypeOptions approx: Bessel | Tschebyscheff | Butterworth | free expression
      mask TypeOptions order: 2 | 3 | 4
      mask TypeOptions vertres: 8 | 12 | 16
      mask Display: disp('DAB')
  DAB - current B : Subsystem  AncestorBlock=elements/DAB  mask(Data Adquisition Board){filter=off, approx=Butterworth, order=2, numerator=[], denominator=[], freq=fCut, resdis=off, vertres=16, xmax=CurrentRange, winsize=WindowSize, G=1.0, fs=fSampling}
      mask prompts: filter "Disable Analog Filter"; approx "Filter approximation"; numerator "Free expression filter: numerator(descending order of s)"; denominator "Free expression filter: denominator:"; freq "Cut-off frequency"; resdis "Disable Vertical Resolution"; vertres "Vertical Resolution: No. of bits"; xmax "Vertical Resolution: signal range"; winsize "Window size"; G "Gain"; fs "Sampling frequency"
      mask help: Performs analog filtering, signal conditioning and sampling. A single signal is the input, a buffer with the signal samples is the output. The options include analog filter enable/disable switch, type, order and cut-off frequency of the analog filter, conditioning gain, sampling frequency, number of bits, the length of the buffer.
      mask init:
      | dab1
      mask Help: web(['file:///' which('dabdoc2.html')]);
      mask TypeOptions approx: Bessel | Tschebyscheff | Butterworth | free expression
      mask TypeOptions order: 2 | 3 | 4
      mask TypeOptions vertres: 8 | 12 | 16
      mask Display: disp('DAB')
  DAB - current C : Subsystem  AncestorBlock=elements/DAB  mask(Data Adquisition Board){filter=off, approx=Butterworth, order=2, numerator=[], denominator=[], freq=fCut, resdis=off, vertres=16, xmax=CurrentRange, winsize=WindowSize, G=1.0, fs=fSampling}
      mask prompts: filter "Disable Analog Filter"; approx "Filter approximation"; numerator "Free expression filter: numerator(descending order of s)"; denominator "Free expression filter: denominator:"; freq "Cut-off frequency"; resdis "Disable Vertical Resolution"; vertres "Vertical Resolution: No. of bits"; xmax "Vertical Resolution: signal range"; winsize "Window size"; G "Gain"; fs "Sampling frequency"
      mask help: Performs analog filtering, signal conditioning and sampling. A single signal is the input, a buffer with the signal samples is the output. The options include analog filter enable/disable switch, type, order and cut-off frequency of the analog filter, conditioning gain, sampling frequency, number of bits, the length of the buffer.
      mask init:
      | dab1
      mask Help: web(['file:///' which('dabdoc2.html')]);
      mask TypeOptions approx: Bessel | Tschebyscheff | Butterworth | free expression
      mask TypeOptions order: 2 | 3 | 4
      mask TypeOptions vertres: 8 | 12 | 16
      mask Display: disp('DAB')
  Demux : Demux  Outputs=3
  Phasor IA : Subsystem  AncestorBlock=powerlib_extras/Measurements/Fourier  DialogController=POWERSYS.PowerSysDialog  mask(Fourier analyser){f1=Freq, n=1}
      mask prompts: f1 "Fundamental frequency f1 (Hz):"; n "Harmonic n (0=DC; 1=fundamental; 2=2nd harm;  ...) :"
      mask help: The Fourier block performs a Fourier analysis of the input signal over a running window of one cycle of the fundamental frequency. First and second outputs return respectively the magnitude and phase (degrees) of the harmonic component specified.
      mask init:
      | k=2-(n==0);
      | power_initmask();
      mask Help: web(psbhelp)
  Phasor IB : Subsystem  AncestorBlock=powerlib_extras/Measurements/Fourier  DialogController=POWERSYS.PowerSysDialog  mask(Fourier analyser){f1=Freq, n=1}
      mask prompts: f1 "Fundamental frequency f1 (Hz):"; n "Harmonic n (0=DC; 1=fundamental; 2=2nd harm;  ...) :"
      mask help: The Fourier block performs a Fourier analysis of the input signal over a running window of one cycle of the fundamental frequency. First and second outputs return respectively the magnitude and phase (degrees) of the harmonic component specified.
      mask init:
      | k=2-(n==0);
      | power_initmask();
      mask Help: web(psbhelp)
  Phasor IC : Subsystem  AncestorBlock=powerlib_extras/Measurements/Fourier  DialogController=POWERSYS.PowerSysDialog  mask(Fourier analyser){f1=Freq, n=1}
      mask prompts: f1 "Fundamental frequency f1 (Hz):"; n "Harmonic n (0=DC; 1=fundamental; 2=2nd harm;  ...) :"
      mask help: The Fourier block performs a Fourier analysis of the input signal over a running window of one cycle of the fundamental frequency. First and second outputs return respectively the magnitude and phase (degrees) of the harmonic component specified.
      mask init:
      | k=2-(n==0);
      | power_initmask();
      mask Help: web(psbhelp)
  Product{,1..3,5} (5 alike) : Product  RndMeth=Zero
  IAf : Outport  InitialOutput=0  VectorParamsAs1DForOutWhenUnconnected=on
  IBf : Outport  Port=2  InitialOutput=0  VectorParamsAs1DForOutWhenUnconnected=on
  ICf : Outport  Port=3  InitialOutput=0  VectorParamsAs1DForOutWhenUnconnected=on
  k0I0f : Outport  Port=4  InitialOutput=0  VectorParamsAs1DForOutWhenUnconnected=on
  iaf : Outport  Port=5  InitialOutput=0  VectorParamsAs1DForOutWhenUnconnected=on
  ibf : Outport  Port=6  InitialOutput=0  VectorParamsAs1DForOutWhenUnconnected=on
  icf : Outport  Port=7  InitialOutput=0  VectorParamsAs1DForOutWhenUnconnected=on
  wires:
  Complex3/1 -> Product5/2
  Product3/1 -> Complex3/2
  Product5/1 -> k0I0f/1
  Add/1 -> Product5/1
  Constant1/1 -> Complex3/1
  Constant2/1 -> Product3/2
  Complex/1 -> Add/1, IAf/1
  Complex2/1 -> Add/3, ICf/1
  Complex1/1 -> Add/2, IBf/1
  Phasor IB/1(magnitude) -> Complex1/1
  Product1/1 -> Complex1/2
  Phasor IC/1(magnitude) -> Complex2/1
  Product2/1 -> Complex2/2
  Product/1 -> Complex/2
  Phasor IA/1(magnitude) -> Complex/1
  Phasor IC/2(angle) -> Product2/1
  Phasor IB/2(angle) -> Product1/1
  Constant/1 -> Product3/1, Product2/2, Product1/2, Product/2
  Phasor IA/2(angle) -> Product/1
  Iabc/1 -> Demux/1
  Demux/1 -> DAB - current A/1(a)
  Demux/3 -> DAB - current C/1(a)
  Demux/2 -> DAB - current B/1(a)
  DAB - current A/1(d) -> iaf/1, Phasor IA/1(signal)
  DAB - current B/1(d) -> Phasor IB/1(signal), ibf/1
  DAB - current C/1(d) -> Phasor IC/1(signal), icf/1

== system Basics/SM_WT1/Impedance Element 1/Impedance Relay Scheme/Analog filtering, signal conditioning/VOLTAGES ==
  Vabc : Inport
  Complex : MagnitudeAngleToComplex
  Complex1 : MagnitudeAngleToComplex
  Complex2 : MagnitudeAngleToComplex
  Constant : Constant  Value=pi/180
  DAB - voltage A : Subsystem  AncestorBlock=elements/DAB  mask(Data Adquisition Board){filter=off, approx=Butterworth, order=2, numerator=[], denominator=[], freq=fCut, resdis=off, vertres=16, xmax=CurrentRange, winsize=WindowSize, G=1.0, fs=fSampling}
      mask prompts: filter "Disable Analog Filter"; approx "Filter approximation"; numerator "Free expression filter: numerator(descending order of s)"; denominator "Free expression filter: denominator:"; freq "Cut-off frequency"; resdis "Disable Vertical Resolution"; vertres "Vertical Resolution: No. of bits"; xmax "Vertical Resolution: signal range"; winsize "Window size"; G "Gain"; fs "Sampling frequency"
      mask help: Performs analog filtering, signal conditioning and sampling. A single signal is the input, a buffer with the signal samples is the output. The options include analog filter enable/disable switch, type, order and cut-off frequency of the analog filter, conditioning gain, sampling frequency, number of bits, the length of the buffer.
      mask init:
      | dab1
      mask Help: web(['file:///' which('dabdoc2.html')]);
      mask TypeOptions approx: Bessel | Tschebyscheff | Butterworth | free expression
      mask TypeOptions order: 2 | 3 | 4
      mask TypeOptions vertres: 8 | 12 | 16
      mask Display: disp('DAB')
  DAB - voltage B : Subsystem  AncestorBlock=elements/DAB  mask(Data Adquisition Board){filter=off, approx=Butterworth, order=2, numerator=[], denominator=[], freq=fCut, resdis=off, vertres=16, xmax=CurrentRange, winsize=WindowSize, G=1.0, fs=fSampling}
      mask prompts: filter "Disable Analog Filter"; approx "Filter approximation"; numerator "Free expression filter: numerator(descending order of s)"; denominator "Free expression filter: denominator:"; freq "Cut-off frequency"; resdis "Disable Vertical Resolution"; vertres "Vertical Resolution: No. of bits"; xmax "Vertical Resolution: signal range"; winsize "Window size"; G "Gain"; fs "Sampling frequency"
      mask help: Performs analog filtering, signal conditioning and sampling. A single signal is the input, a buffer with the signal samples is the output. The options include analog filter enable/disable switch, type, order and cut-off frequency of the analog filter, conditioning gain, sampling frequency, number of bits, the length of the buffer.
      mask init:
      | dab1
      mask Help: web(['file:///' which('dabdoc2.html')]);
      mask TypeOptions approx: Bessel | Tschebyscheff | Butterworth | free expression
      mask TypeOptions order: 2 | 3 | 4
      mask TypeOptions vertres: 8 | 12 | 16
      mask Display: disp('DAB')
  DAB - voltage C : Subsystem  AncestorBlock=elements/DAB  mask(Data Adquisition Board){filter=off, approx=Butterworth, order=2, numerator=[], denominator=[], freq=fCut, resdis=off, vertres=16, xmax=CurrentRange, winsize=WindowSize, G=1.0, fs=fSampling}
      mask prompts: filter "Disable Analog Filter"; approx "Filter approximation"; numerator "Free expression filter: numerator(descending order of s)"; denominator "Free expression filter: denominator:"; freq "Cut-off frequency"; resdis "Disable Vertical Resolution"; vertres "Vertical Resolution: No. of bits"; xmax "Vertical Resolution: signal range"; winsize "Window size"; G "Gain"; fs "Sampling frequency"
      mask help: Performs analog filtering, signal conditioning and sampling. A single signal is the input, a buffer with the signal samples is the output. The options include analog filter enable/disable switch, type, order and cut-off frequency of the analog filter, conditioning gain, sampling frequency, number of bits, the length of the buffer.
      mask init:
      | dab1
      mask Help: web(['file:///' which('dabdoc2.html')]);
      mask TypeOptions approx: Bessel | Tschebyscheff | Butterworth | free expression
      mask TypeOptions order: 2 | 3 | 4
      mask TypeOptions vertres: 8 | 12 | 16
      mask Display: disp('DAB')
  Demux : Demux  Outputs=3
  Phasor VA : Subsystem  AncestorBlock=powerlib_extras/Measurements/Fourier  DialogController=POWERSYS.PowerSysDialog  mask(Fourier analyser){f1=Freq, n=1}
      mask prompts: f1 "Fundamental frequency f1 (Hz):"; n "Harmonic n (0=DC; 1=fundamental; 2=2nd harm;  ...) :"
      mask help: The Fourier block performs a Fourier analysis of the input signal over a running window of one cycle of the fundamental frequency. First and second outputs return respectively the magnitude and phase (degrees) of the harmonic component specified.
      mask init:
      | k=2-(n==0);
      | power_initmask();
      mask Help: web(psbhelp)
  Phasor VB : Subsystem  AncestorBlock=powerlib_extras/Measurements/Fourier  DialogController=POWERSYS.PowerSysDialog  mask(Fourier analyser){f1=Freq, n=1}
      mask prompts: f1 "Fundamental frequency f1 (Hz):"; n "Harmonic n (0=DC; 1=fundamental; 2=2nd harm;  ...) :"
      mask help: The Fourier block performs a Fourier analysis of the input signal over a running window of one cycle of the fundamental frequency. First and second outputs return respectively the magnitude and phase (degrees) of the harmonic component specified.
      mask init:
      | k=2-(n==0);
      | power_initmask();
      mask Help: web(psbhelp)
  Phasor VC : Subsystem  AncestorBlock=powerlib_extras/Measurements/Fourier  DialogController=POWERSYS.PowerSysDialog  mask(Fourier analyser){f1=Freq, n=1}
      mask prompts: f1 "Fundamental frequency f1 (Hz):"; n "Harmonic n (0=DC; 1=fundamental; 2=2nd harm;  ...) :"
      mask help: The Fourier block performs a Fourier analysis of the input signal over a running window of one cycle of the fundamental frequency. First and second outputs return respectively the magnitude and phase (degrees) of the harmonic component specified.
      mask init:
      | k=2-(n==0);
      | power_initmask();
      mask Help: web(psbhelp)
  Product : Product  RndMeth=Zero
  Product1 : Product  RndMeth=Zero
  Product2 : Product  RndMeth=Zero
  VAf : Outport  InitialOutput=0  VectorParamsAs1DForOutWhenUnconnected=on
  VBf : Outport  Port=2  InitialOutput=0  VectorParamsAs1DForOutWhenUnconnected=on
  VCf : Outport  Port=3  InitialOutput=0  VectorParamsAs1DForOutWhenUnconnected=on
  vaf : Outport  Port=4  InitialOutput=0  VectorParamsAs1DForOutWhenUnconnected=on
  vbf : Outport  Port=5  InitialOutput=0  VectorParamsAs1DForOutWhenUnconnected=on
  vcf : Outport  Port=6  InitialOutput=0  VectorParamsAs1DForOutWhenUnconnected=on
  wires:
  Complex/1 -> VAf/1
  Complex2/1 -> VCf/1
  Complex1/1 -> VBf/1
  Phasor VB/1(magnitude) -> Complex1/1
  Product1/1 -> Complex1/2
  Phasor VC/1(magnitude) -> Complex2/1
  Product2/1 -> Complex2/2
  Product/1 -> Complex/2
  Phasor VA/1(magnitude) -> Complex/1
  Phasor VC/2(angle) -> Product2/1
  Phasor VB/2(angle) -> Product1/1
  Constant/1 -> Product2/2, Product1/2, Product/2
  Phasor VA/2(angle) -> Product/1
  DAB - voltage C/1(d) -> Phasor VC/1(signal), vcf/1
  DAB - voltage B/1(d) -> Phasor VB/1(signal), vbf/1
  DAB - voltage A/1(d) -> vaf/1, Phasor VA/1(signal)
  Demux/2 -> DAB - voltage B/1(a)
  Demux/3 -> DAB - voltage C/1(a)
  Demux/1 -> DAB - voltage A/1(a)
  Vabc/1 -> Demux/1

== system Basics/SM_WT1/Impedance Element 1/Impedance Relay Scheme/Fault A-B-C Measurement/Zone 1 ==
  Z : Inport
  <V : Inport  Port=2
  " 5" : Fcn  Expr=sqrt(u)
  " 6" : RelationalOperator  Operator=<  OutDataTypeStr=boolean  RndMeth=Nearest
  6 : Fcn  Expr=sqrt(u)
  Integrator : Integrator
  Product{,1..3} (4 alike) : Product  RndMeth=Zero
  "R, X" : Demux  Outputs=2
  Rdiff : Sum  Inputs=+-  SaturateOnIntegerOverflow=on  InputSameDT=on  OutDataTypeStr=Inherit: Same as first input
  Rr : Constant  Value=Rr/2
  Startup : Product  Inputs=3  RndMeth=Zero
  Step : Step  Time=0.017  SampleTime=0
  TRIP output contact : Relay  OnSwitchValue=0.9999  OffSwitchValue=-1
  Xdiff : Sum  Inputs=+-  SaturateOnIntegerOverflow=on  InputSameDT=on  OutDataTypeStr=Inherit: Same as first input
  Xr : Constant  Value=Xr/2
  Zm2 : Sum  SaturateOnIntegerOverflow=on  InputSameDT=on  OutDataTypeStr=Inherit: Same as first input
  Zr2 : Sum  SaturateOnIntegerOverflow=on  InputSameDT=on  OutDataTypeStr=Inherit: Same as first input
  delay : RelationalOperator  Operator=>  RndMeth=Nearest  InputSameDT=on
  time delay : Constant  Value=Td+0.001
  TRIP : Outport  InitialOutput=0  VectorParamsAs1DForOutWhenUnconnected=on
  Zm : Outport  Port=2  InitialOutput=0  VectorParamsAs1DForOutWhenUnconnected=on
  Zr : Outport  Port=3  InitialOutput=0  VectorParamsAs1DForOutWhenUnconnected=on
  wires:
  Z/1 -> "R, X"/1
  Rr/1 -> Rdiff/1, Product1/2, Product1/1
  "R, X"/1 -> Rdiff/2
  "R, X"/2 -> Xdiff/1
  Xr/1 -> Xdiff/2, Product3/2, Product3/1
  Xdiff/1 -> Product2/2, Product2/1
  Product/1 -> Zm2/1
  Product2/1 -> Zm2/2
  Product1/1 -> Zr2/1
  Product3/1 -> Zr2/2
  Zm2/1 -> 6/1
  Zr2/1 -> " 5"/1
  6/1 -> " 6"/1, Zm/1
  " 5"/1 -> " 6"/2, Zr/1
  " 6"/1 -> Startup/1
  <V/1 -> Startup/3
  Step/1 -> Startup/2
  Rdiff/1 -> Product/1, Product/2
  Integrator/1 -> delay/1
  time delay/1 -> delay/2
  delay/1 -> TRIP output contact/1
  Startup/1 -> Integrator/1
  TRIP output contact/1 -> TRIP/1

== system Basics/SM_WT1/Impedance Element 1/Impedance Relay Scheme/Fault A-B-C Measurement/Zone 2 ==
  Z : Inport
  <V : Inport  Port=2
  " 5" : Fcn  Expr=sqrt(u)
  " 6" : RelationalOperator  Operator=<  OutDataTypeStr=boolean  RndMeth=Nearest
  6 : Fcn  Expr=sqrt(u)
  Integrator : Integrator
  Product{,1..3} (4 alike) : Product  RndMeth=Zero
  "R, X" : Demux  Outputs=2
  Rdiff : Sum  Inputs=+-  SaturateOnIntegerOverflow=on  InputSameDT=on  OutDataTypeStr=Inherit: Same as first input
  Rr : Constant  Value=Rr/2
  Startup : Product  Inputs=3  RndMeth=Zero
  Step : Step  Time=0.017  SampleTime=0
  TRIP output contact : Relay  OnSwitchValue=0.9999  OffSwitchValue=-1
  Xdiff : Sum  Inputs=+-  SaturateOnIntegerOverflow=on  InputSameDT=on  OutDataTypeStr=Inherit: Same as first input
  Xr : Constant  Value=Xr/2
  Zm2 : Sum  SaturateOnIntegerOverflow=on  InputSameDT=on  OutDataTypeStr=Inherit: Same as first input
  Zr2 : Sum  SaturateOnIntegerOverflow=on  InputSameDT=on  OutDataTypeStr=Inherit: Same as first input
  delay : RelationalOperator  Operator=>  RndMeth=Nearest  InputSameDT=on
  time delay : Constant  Value=Td+0.001
  TRIP : Outport  InitialOutput=0  VectorParamsAs1DForOutWhenUnconnected=on
  Zm : Outport  Port=2  InitialOutput=0  VectorParamsAs1DForOutWhenUnconnected=on
  Zr : Outport  Port=3  InitialOutput=0  VectorParamsAs1DForOutWhenUnconnected=on
  wires:
  TRIP output contact/1 -> TRIP/1
  Startup/1 -> Integrator/1
  delay/1 -> TRIP output contact/1
  time delay/1 -> delay/2
  Integrator/1 -> delay/1
  Rdiff/1 -> Product/2, Product/1
  Step/1 -> Startup/2
  <V/1 -> Startup/3
  " 6"/1 -> Startup/1
  " 5"/1 -> Zr/1, " 6"/2
  6/1 -> Zm/1, " 6"/1
  Zr2/1 -> " 5"/1
  Zm2/1 -> 6/1
  Product3/1 -> Zr2/2
  Product1/1 -> Zr2/1
  Product2/1 -> Zm2/2
  Product/1 -> Zm2/1
  Xdiff/1 -> Product2/1, Product2/2
  Xr/1 -> Product3/1, Product3/2, Xdiff/2
  "R, X"/2 -> Xdiff/1
  "R, X"/1 -> Rdiff/2
  Rr/1 -> Product1/1, Product1/2, Rdiff/1
  Z/1 -> "R, X"/1
